simulink model "sampleModel2027"  (R2023a)
settings: Solver=VariableStepAuto  StartTime=0.0  StopTime=10.0  RelTol=1e-3
libraries: hdlsllib x5, simulink x2
settings Model: Creator=user1  LastModifiedBy=user1

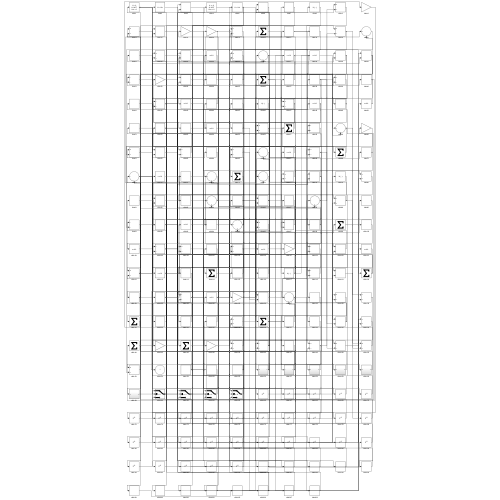
[thumbnail: Simulink's stored preview of the top-level diagram]
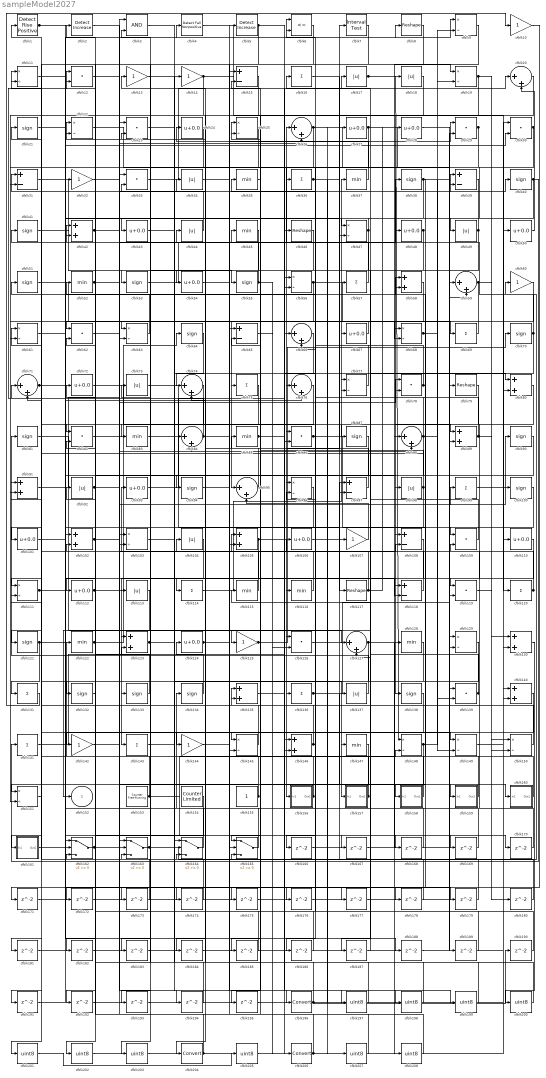
== system sampleModel2027 ==
  cfblk1 : hdlsllib/Logic and Bit Operations/Detect Rise Positive  vinit=0  OutDataTypeStr=boolean
  cfblk{10,13..14,32,60,107,125,142,144} (9 alike) : Gain
  cfblk{21,38,40..41,51,53,55,64,70,81,87,90,94,100,121,132..134,138} (19 alike) : Signum
  cfblk{24,27..28,43,48,50,54,67,72,93,101,106,110,112,124} (15 alike) : Bias  Bias=0.0  SaturateOnIntegerOverflow=off
  cfblk{42,58,80,89,91,102,105,123,130,135,140,146} (12 alike) : Sum
  cfblk{9,11,19,22,25,47,56,61,63,68,77,96,103,111,129,145,148..151} (20 alike) : Product  Inputs=*/  RndMeth=Zero  SaturateOnIntegerOverflow=on
  cfblk{17..18,34,44,49,73,92,98,104,113,137} (11 alike) : Abs  SaturateOnIntegerOverflow=off
  cfblk{15,31,39,65,97,108,118} (7 alike) : Sum  Inputs=+-
  cfblk{12,23,29..30,33,62,78,82,86,109,119,126,139} (13 alike) : DotProduct  OutDataTypeStr=Inherit: Inherit via internal rule
  cfblk{16,36,57,69,75,99,114,120,131,136,141,143} (12 alike) : Sum  Inputs=+
  cfblk{35,37,45,52,83,85,115..116,122,128,147} (11 alike) : MinMax
  cfblk{8,46,79,117} (4 alike) : Reshape
  cfblk{20,26,59,66,71,74,76,84,88,95,127} (11 alike) : Sum  Inputs=|++
  cfblk153 : hdlsllib/Sources/Counter Free-Running  NumBits=16  tsamp=-1
  cfblk154 : hdlsllib/Sources/Counter Limited  uplimit=7  tsamp=-1
  cfblk155 : Constant  SampleTime=-1
  cfblk156 : Subsystem
      settings: LibrarySourceBlock=|
      | hdlsllib/Ports &
      | Subsystems/Subsystem
  cfblk157 : Subsystem
      settings: LibrarySourceBlock=|
      | hdlsllib/Ports &
      | Subsystems/Subsystem
  cfblk158 : Subsystem
      settings: LibrarySourceBlock=|
      | hdlsllib/Ports &
      | Subsystems/Subsystem
  cfblk159 : Subsystem
      settings: LibrarySourceBlock=|
      | hdlsllib/Ports &
      | Subsystems/Subsystem
  cfblk160 : Subsystem
      settings: LibrarySourceBlock=|
      | hdlsllib/Ports &
      | Subsystems/Subsystem
  cfblk161 : Subsystem
      settings: LibrarySourceBlock=|
      | hdlsllib/Ports &
      | Subsystems/Subsystem
  cfblk{162..165} (4 alike) : Switch  SaturateOnIntegerOverflow=off  InputSameDT=off
  cfblk{166..195} (30 alike) : Delay  SampleTime=1
  cfblk196 : DataTypeConversion  SaturateOnIntegerOverflow=off  RndMeth=Floor
  cfblk{197..203,205,207..208} (10 alike) : DataTypeConversion  OutDataTypeStr=uint8  SaturateOnIntegerOverflow=off  RndMeth=Floor
  cfblk2 : simulink/Logic and Bit Operations/Detect Increase  vinit=0.0  OutDataTypeStr=boolean
      settings: LibrarySourceBlock=|
      | hdlsllib/Logic and Bit
      | Operations/Detect
      | Increase
  cfblk204 : DataTypeConversion  SaturateOnIntegerOverflow=off  RndMeth=Floor
  cfblk206 : DataTypeConversion  SaturateOnIntegerOverflow=off  RndMeth=Floor
  cfblk3 : Logic  AllPortsSameDT=off  OutDataTypeStr=boolean
  cfblk4 : hdlsllib/Logic and Bit Operations/Detect Fall Nonpositive  vinit=0  OutDataTypeStr=boolean
  cfblk5 : simulink/Logic and Bit Operations/Detect Increase  vinit=0.0  OutDataTypeStr=boolean
      settings: LibrarySourceBlock=|
      | hdlsllib/Logic and Bit
      | Operations/Detect
      | Increase
  cfblk6 : RelationalOperator  Operator=<=  OutDataTypeStr=boolean  InputSameDT=off
  cfblk7 : hdlsllib/Logic and Bit Operations/Interval Test  IntervalClosedRight=on  uplimit=0.5  IntervalClosedLeft=on  lowlimit=-0.5  OutDataTypeStr=boolean
  cfblk152 : Outport  VectorParamsAs1DForOutWhenUnconnected=off
  wires:
  cfblk146/1 -> cfblk135/1, cfblk66/2
  cfblk156/1(Out1) -> cfblk122/1, cfblk71/2
  cfblk129/1 -> cfblk157/1(In1)
  cfblk119/1 -> cfblk130/1
  cfblk77/1 -> cfblk51/1
  cfblk56/1 -> cfblk152/1, cfblk151/2
  cfblk33/1 -> cfblk20/1
  cfblk59/1 -> cfblk95/1, cfblk180/1
  cfblk110/1 -> cfblk204/1
  cfblk46/1 -> cfblk156/1(In1)
  cfblk69/1 -> cfblk62/1
  cfblk84/1 -> cfblk12/1, cfblk198/1
  cfblk52/1 -> cfblk118/2, cfblk194/1
  cfblk47/1 -> cfblk43/1, cfblk185/1, cfblk186/1
  cfblk81/1 -> cfblk136/1
  cfblk17/1 -> cfblk148/1, cfblk19/1
  cfblk57/1 -> cfblk26/1
  cfblk132/1 -> cfblk72/1
  cfblk135/1 -> cfblk17/1
  cfblk114/1 -> cfblk37/1
  cfblk31/1 -> cfblk55/1
  cfblk125/1 -> cfblk70/1, cfblk78/1
  cfblk159/1(Out1) -> cfblk25/1
  cfblk26/1 -> cfblk86/1, cfblk59/1, cfblk181/1
  cfblk95/1 -> cfblk13/1, cfblk94/1
  cfblk91/1 -> cfblk33/1
  cfblk105/1 -> cfblk7/1, cfblk113/1
  cfblk98/1 -> cfblk25/2, cfblk61/1, cfblk174/1
  cfblk79/1 -> cfblk138/1
  cfblk106/1 -> cfblk107/1
  cfblk163/1 -> cfblk60/1, cfblk99/1
  cfblk67/1 -> cfblk63/1
  cfblk112/1 -> cfblk64/1, cfblk56/1
  cfblk165/1 -> cfblk92/1
  cfblk107/1 -> cfblk95/2
  cfblk4/1 -> cfblk128/1
  cfblk164/1 -> cfblk134/1
  cfblk117/1 -> cfblk93/1, cfblk28/1
  cfblk40/1 -> cfblk141/1, cfblk56/2
  cfblk62/1 -> cfblk44/1
  cfblk66/1 -> cfblk86/2
  cfblk73/1 -> cfblk117/1
  cfblk148/1 -> cfblk19/2, cfblk166/1
  cfblk65/1 -> cfblk206/1
  cfblk14/1 -> cfblk120/1, cfblk61/2
  cfblk118/1 -> cfblk67/1
  cfblk151/1 -> cfblk71/1
  cfblk121/1 -> cfblk131/1, cfblk58/2, cfblk11/2
  cfblk137/1 -> cfblk81/1
  cfblk90/1 -> cfblk112/1
  cfblk141/1 -> cfblk46/1
  cfblk136/1 -> cfblk18/1, cfblk159/1(In1)
  cfblk20/1 -> cfblk114/1
  cfblk145/1 -> cfblk91/1
  cfblk85/1 -> cfblk147/1, cfblk197/1
  cfblk124/1 -> cfblk5/1, cfblk106/1
  cfblk89/1 -> cfblk41/1, cfblk150/2
  cfblk83/1 -> cfblk14/1
  cfblk157/1(Out1) -> cfblk34/1, cfblk82/2
  cfblk70/1 -> cfblk45/1, cfblk177/1
  cfblk43/1 -> cfblk75/1
  cfblk37/1 -> cfblk24/1
  cfblk42/1 -> cfblk40/1, cfblk160/1(In1)
  cfblk153/1 -> cfblk148/2, cfblk111/2, cfblk208/1
  cfblk131/1 -> cfblk10/1
  cfblk63/1 -> cfblk21/1
  cfblk139/1 -> cfblk115/1, cfblk16/1
  cfblk100/1 -> cfblk109/1
  cfblk22/1 -> cfblk129/2
  cfblk32/1 -> cfblk4/1
  cfblk29/1 -> cfblk121/1, cfblk173/1
  cfblk126/1 -> cfblk79/1
  cfblk12/1 -> cfblk163/1
  cfblk50/1 -> cfblk20/2
  cfblk27/1 -> cfblk165/1, cfblk39/2
  cfblk60/1 -> cfblk165/2
  cfblk41/1 -> cfblk53/1
  cfblk30/1 -> cfblk126/1, cfblk31/2, cfblk49/1
  cfblk23/1 -> cfblk96/1
  cfblk120/1 -> cfblk105/1, cfblk52/1
  cfblk138/1 -> cfblk145/1
  cfblk15/1 -> cfblk132/1
  cfblk39/1 -> cfblk76/1
  cfblk8/1 -> cfblk105/2
  cfblk102/1 -> cfblk88/2, cfblk26/2
  cfblk161/1(Out1) -> cfblk57/1
  cfblk86/1 -> cfblk139/1, cfblk176/1
  cfblk123/1 -> cfblk84/2, cfblk168/1
  cfblk158/1(Out1) -> cfblk6/1
  cfblk38/1 -> cfblk158/1(In1), cfblk42/2, cfblk149/2, cfblk59/2
  cfblk51/1 -> cfblk146/2
  cfblk61/1 -> cfblk32/1
  cfblk36/1 -> cfblk118/1, cfblk207/1
  cfblk150/1 -> cfblk42/1
  cfblk96/1 -> cfblk162/2
  cfblk44/1 -> cfblk31/1
  cfblk128/1 -> cfblk142/1
  cfblk49/1 -> cfblk47/1, cfblk187/1
  cfblk122/1 -> cfblk68/1, cfblk108/2
  cfblk53/1 -> cfblk38/1
  cfblk82/1 -> cfblk87/1
  cfblk88/1 -> cfblk35/1, cfblk9/2, cfblk193/1
  cfblk71/1 -> cfblk111/1, cfblk145/2, cfblk116/1, cfblk188/1
  cfblk101/1 -> cfblk9/1
  cfblk25/1 -> cfblk144/1
  cfblk142/1 -> cfblk63/2
  cfblk1/1 -> cfblk97/2, cfblk69/1, cfblk47/2
  cfblk34/1 -> cfblk80/1
  cfblk134/1 -> cfblk124/1
  cfblk108/1 -> cfblk143/1
  cfblk144/1 -> cfblk29/1
  cfblk104/1 -> cfblk164/2
  cfblk74/1 -> cfblk101/1
  cfblk143/1 -> cfblk48/1
  cfblk149/1 -> cfblk50/1
  cfblk99/1 -> cfblk90/1
  cfblk72/1 -> cfblk89/1
  cfblk35/1 -> cfblk15/2
  cfblk160/1(Out1) -> cfblk58/1
  cfblk97/1 -> cfblk22/1
  cfblk162/1 -> cfblk100/1, cfblk8/1
  cfblk55/1 -> cfblk33/2, cfblk126/2
  cfblk45/1 -> cfblk54/1
  cfblk155/1 -> cfblk23/2, cfblk151/1
  cfblk5/1 -> cfblk133/1, cfblk68/2, cfblk83/1
  cfblk9/1 -> cfblk82/1
  cfblk133/1 -> cfblk102/2
  cfblk92/1 -> cfblk127/1, cfblk78/2
  cfblk19/1 -> cfblk103/2, cfblk150/1
  cfblk80/1 -> cfblk119/1
  cfblk109/1 -> cfblk77/1
  cfblk48/1 -> cfblk123/1, cfblk74/2
  cfblk64/1 -> cfblk74/1
  cfblk13/1 -> cfblk137/1
  cfblk18/1 -> cfblk125/1
  cfblk116/1 -> cfblk73/1
  cfblk58/1 -> cfblk91/2
  cfblk54/1 -> cfblk149/1
  cfblk3/1 -> cfblk196/1
  cfblk111/1 -> cfblk76/2, cfblk30/2
  cfblk127/1 -> cfblk161/1(In1), cfblk169/1
  cfblk16/1 -> cfblk98/1
  cfblk93/1 -> cfblk39/1
  cfblk68/1 -> cfblk108/1, cfblk139/2
  cfblk78/1 -> cfblk36/1, cfblk178/1
  cfblk115/1 -> cfblk11/1
  cfblk166/1 -> cfblk88/1
  cfblk103/1 -> cfblk167/1
  cfblk167/1 -> cfblk129/1
  cfblk168/1 -> cfblk102/1
  cfblk169/1 -> cfblk123/2
  cfblk11/1 -> cfblk170/1
  cfblk170/1 -> cfblk109/2
  cfblk10/1 -> cfblk171/1
  cfblk171/1 -> cfblk146/1
  cfblk24/1 -> cfblk172/1
  cfblk172/1 -> cfblk29/2
  cfblk173/1 -> cfblk162/3
  cfblk174/1 -> cfblk164/3
  cfblk21/1 -> cfblk175/1
  cfblk175/1 -> cfblk135/2
  cfblk176/1 -> cfblk96/2
  cfblk177/1 -> cfblk127/2
  cfblk178/1 -> cfblk12/2
  cfblk94/1 -> cfblk179/1
  cfblk179/1 -> cfblk97/1
  cfblk180/1 -> cfblk1/1
  cfblk181/1 -> cfblk130/2
  cfblk87/1 -> cfblk182/1
  cfblk182/1 -> cfblk84/1
  cfblk76/1 -> cfblk183/1
  cfblk183/1 -> cfblk89/2
  cfblk75/1 -> cfblk184/1
  cfblk184/1 -> cfblk30/1
  cfblk185/1 -> cfblk163/2
  cfblk186/1 -> cfblk163/3
  cfblk187/1 -> cfblk77/2
  cfblk188/1 -> cfblk119/2
  cfblk28/1 -> cfblk189/1
  cfblk189/1 -> cfblk22/2
  cfblk190/1 -> cfblk6/2
  cfblk7/1 -> cfblk191/1
  cfblk191/1 -> cfblk162/1
  cfblk113/1 -> cfblk192/1
  cfblk192/1 -> cfblk15/1
  cfblk193/1 -> cfblk80/2
  cfblk194/1 -> cfblk164/1
  cfblk147/1 -> cfblk195/1
  cfblk195/1 -> cfblk85/1
  cfblk196/1 -> cfblk190/1, cfblk27/1, cfblk165/3
  cfblk197/1 -> cfblk3/1
  cfblk198/1 -> cfblk3/2
  cfblk2/1 -> cfblk199/1
  cfblk199/1 -> cfblk104/1
  cfblk130/1 -> cfblk200/1
  cfblk200/1 -> cfblk2/1
  cfblk140/1 -> cfblk201/1
  cfblk154/1 -> cfblk202/1
  cfblk202/1 -> cfblk140/1
  cfblk6/1 -> cfblk203/1
  cfblk203/1 -> cfblk140/2
  cfblk204/1 -> cfblk66/1, cfblk23/1
  cfblk201/1 -> cfblk205/1
  cfblk205/1 -> cfblk110/1
  cfblk206/1 -> cfblk62/2, cfblk103/1
  cfblk207/1 -> cfblk65/1
  cfblk208/1 -> cfblk65/2

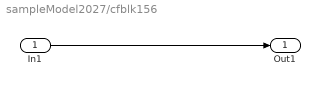
== system sampleModel2027/cfblk156 ==
  In1 : Inport
  Out1 : Outport
  wires:
  In1/1 -> Out1/1

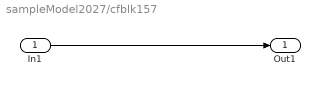
== system sampleModel2027/cfblk157 ==
  In1 : Inport
  Out1 : Outport
  wires:
  In1/1 -> Out1/1

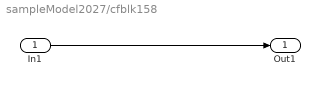
== system sampleModel2027/cfblk158 ==
  In1 : Inport
  Out1 : Outport
  wires:
  In1/1 -> Out1/1

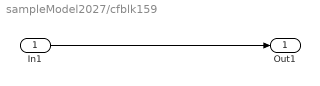
== system sampleModel2027/cfblk159 ==
  In1 : Inport
  Out1 : Outport
  wires:
  In1/1 -> Out1/1

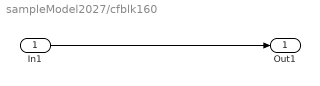
== system sampleModel2027/cfblk160 ==
  In1 : Inport
  Out1 : Outport
  wires:
  In1/1 -> Out1/1

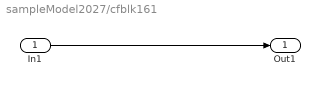
== system sampleModel2027/cfblk161 ==
  In1 : Inport
  Out1 : Outport
  wires:
  In1/1 -> Out1/1
